simulink model "d_014_dyn_l10"  (Simulink 5.1)
settings: Solver=ode45  StartTime=0.0  StopTime=10.0  RelTol=1e-3
libraries: fm_lib x24
(part 2 of 2)

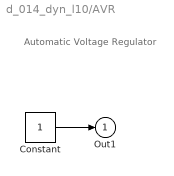
== system d_014_dyn_l10/AVR ==
  note: Automatic Voltage Regulator
  Constant : Constant  OutDataType=sfix(16)  OutScaling=2^0
  Out1 : Outport
  wires:
  Constant/1 -> Out1/1

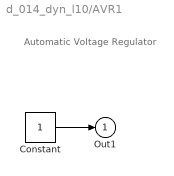
== system d_014_dyn_l10/AVR1 ==
  note: Automatic Voltage Regulator
  Constant : Constant  OutDataType=sfix(16)  OutScaling=2^0
  Out1 : Outport
  wires:
  Constant/1 -> Out1/1

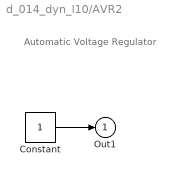
== system d_014_dyn_l10/AVR2 ==
  note: Automatic Voltage Regulator
  Constant : Constant  OutDataType=sfix(16)  OutScaling=2^0
  Out1 : Outport
  wires:
  Constant/1 -> Out1/1

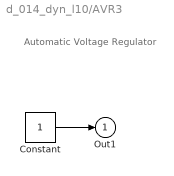
== system d_014_dyn_l10/AVR3 ==
  note: Automatic Voltage Regulator
  Constant : Constant  OutDataType=sfix(16)  OutScaling=2^0
  Out1 : Outport
  wires:
  Constant/1 -> Out1/1

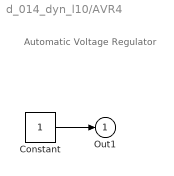
== system d_014_dyn_l10/AVR4 ==
  note: Automatic Voltage Regulator
  Constant : Constant  OutDataType=sfix(16)  OutScaling=2^0
  Out1 : Outport
  wires:
  Constant/1 -> Out1/1

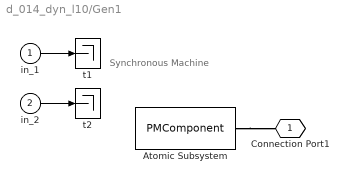
== system d_014_dyn_l10/Gen1 ==
  note: Synchronous Machine
  in_1 : Inport  OutDataType=sfix(16)  OutScaling=2^0
  in_2 : Inport  Port=2  OutDataType=sfix(16)  OutScaling=2^0
  Atomic Subsystem : PMComponent  PhysicalDomain=psatdomain  LeftPortType=p1  RightPortType=p1  RConnTagsString=__newr0
  t1 : Terminator
  t2 : Terminator
  Connection Port1 : PMIOPort  Tag=PMCPort  Orientation=left  Port=1  Side=Right
  wires:
  in_1/1 -> t1/1
  in_2/1 -> t2/1
  connections:
  Atomic Subsystem/RConn1 -- Connection Port1/RConn1

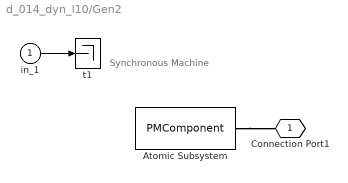
== system d_014_dyn_l10/Gen2 ==
  note: Synchronous Machine
  in_1 : Inport  OutDataType=sfix(16)  OutScaling=2^0
  Atomic Subsystem : PMComponent  PhysicalDomain=psatdomain  LeftPortType=p1  RightPortType=p1  RConnTagsString=__newr0
  t1 : Terminator
  Connection Port1 : PMIOPort  Tag=PMCPort  Orientation=left  Port=1  Side=Right
  wires:
  in_1/1 -> t1/1
  connections:
  Atomic Subsystem/RConn1 -- Connection Port1/RConn1

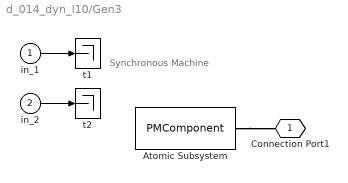
== system d_014_dyn_l10/Gen3 ==
  note: Synchronous Machine
  in_1 : Inport  OutDataType=sfix(16)  OutScaling=2^0
  in_2 : Inport  Port=2  OutDataType=sfix(16)  OutScaling=2^0
  Atomic Subsystem : PMComponent  PhysicalDomain=psatdomain  LeftPortType=p1  RightPortType=p1  RConnTagsString=__newr0
  t1 : Terminator
  t2 : Terminator
  Connection Port1 : PMIOPort  Tag=PMCPort  Orientation=left  Port=1  Side=Right
  wires:
  in_1/1 -> t1/1
  in_2/1 -> t2/1
  connections:
  Atomic Subsystem/RConn1 -- Connection Port1/RConn1

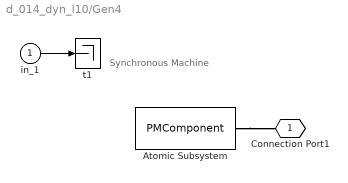
== system d_014_dyn_l10/Gen4 ==
  note: Synchronous Machine
  in_1 : Inport  OutDataType=sfix(16)  OutScaling=2^0
  Atomic Subsystem : PMComponent  PhysicalDomain=psatdomain  LeftPortType=p1  RightPortType=p1  RConnTagsString=__newr0
  t1 : Terminator
  Connection Port1 : PMIOPort  Tag=PMCPort  Orientation=left  Port=1  Side=Right
  wires:
  in_1/1 -> t1/1
  connections:
  Atomic Subsystem/RConn1 -- Connection Port1/RConn1

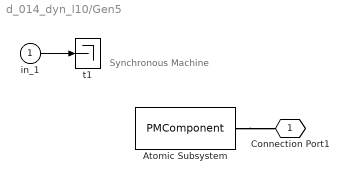
== system d_014_dyn_l10/Gen5 ==
  note: Synchronous Machine
  in_1 : Inport  OutDataType=sfix(16)  OutScaling=2^0
  Atomic Subsystem : PMComponent  PhysicalDomain=psatdomain  LeftPortType=p1  RightPortType=p1  RConnTagsString=__newr0
  t1 : Terminator
  Connection Port1 : PMIOPort  Tag=PMCPort  Orientation=left  Port=1  Side=Right
  wires:
  in_1/1 -> t1/1
  connections:
  Atomic Subsystem/RConn1 -- Connection Port1/RConn1

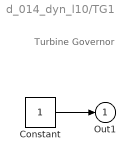
== system d_014_dyn_l10/TG1 ==
  note: Turbine Governor
  Constant : Constant  OutDataType=sfix(16)  OutScaling=2^0
  Out1 : Outport
  wires:
  Constant/1 -> Out1/1

== system d_014_dyn_l10/TG2 ==
  note: Turbine Governor
  Constant : Constant  OutDataType=sfix(16)  OutScaling=2^0
  Out1 : Outport
  wires:
  Constant/1 -> Out1/1
